simulink model "Example"  (Simulink 7.3)
settings: Solver=ode45  StartTime=10  StopTime=3600  RelTol=1e-3
libraries: simulink x2
settings Model: Creator=admin  LastModifiedBy=admin

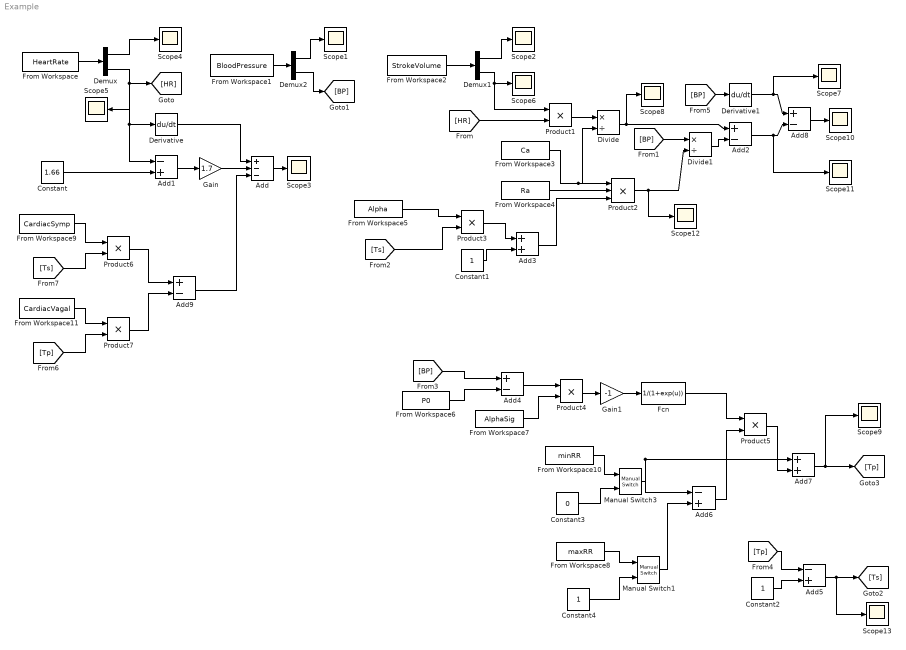
== system Example ==
  Add : Sum  Inputs=+--  OutDataType=fixdt(1, 16)  OutScaling=2^-10
  Add1 : Sum  Inputs=-+  OutDataType=fixdt(1, 16)  OutScaling=2^-10
  Add{2,4,8..9} (4 alike) : Sum  Inputs=+-  OutDataType=fixdt(1, 16)  OutScaling=2^-10
  Add3 : Sum  OutDataType=fixdt(1, 16)  OutScaling=2^-10
  Add5 : Sum  Inputs=-+  OutDataType=fixdt(1, 16)  OutScaling=2^-10
  Add6 : Sum  Inputs=-+  OutDataType=fixdt(1, 16)  OutScaling=2^-10
  Add7 : Sum  OutDataType=fixdt(1, 16)  OutScaling=2^-10
  Constant : Constant  Value=1.66  OutDataType=fixdt(1, 16)  OutScaling=2^0
  Constant1 : Constant  OutDataType=fixdt(1, 16)  OutScaling=2^0
  Constant2 : Constant  OutDataType=fixdt(1, 16)  OutScaling=2^0
  Constant3 : Constant  Value=0  OutDataType=fixdt(1, 16)  OutScaling=2^0
  Constant4 : Constant  OutDataType=fixdt(1, 16)  OutScaling=2^0
  Demux : Demux  Outputs=2
  Demux1 : Demux  Outputs=2
  Demux2 : Demux  Outputs=2
  Derivative : Derivative
  Derivative1 : Derivative
  Divide : Product  Inputs=*/  OutDataType=fixdt(1, 16)  OutScaling=2^-10
  Divide1 : Product  Inputs=*/  OutDataType=fixdt(1, 16)  OutScaling=2^-10
  Fcn : Fcn  Expr=1/(1+exp(u))
  From Workspace : FromWorkspace  VariableName=HeartRate  SampleTime=1
  From Workspace1 : FromWorkspace  VariableName=BloodPressure  SampleTime=1
  From Workspace10 : FromWorkspace  VariableName=minRR  SampleTime=0
  From Workspace11 : FromWorkspace  VariableName=CardiacVagal  SampleTime=1
  From Workspace2 : FromWorkspace  VariableName=StrokeVolume  SampleTime=1
  From Workspace3 : FromWorkspace  VariableName=Ca  SampleTime=0
  From Workspace4 : FromWorkspace  VariableName=Ra  SampleTime=0
  From Workspace5 : FromWorkspace  VariableName=Alpha  SampleTime=0
  From Workspace6 : FromWorkspace  VariableName=P0  SampleTime=0
  From Workspace7 : FromWorkspace  VariableName=AlphaSig  SampleTime=0
  From Workspace8 : FromWorkspace  VariableName=maxRR  SampleTime=0
  From Workspace9 : FromWorkspace  VariableName=CardiacSymp  SampleTime=1
  Gain : Gain  Gain=1.7  ParameterDataType=fixdt(1, 16)  ParameterScaling=2^0  OutDataType=fixdt(1, 16)  OutScaling=2^0
  Gain1 : Gain  Gain=-1  ParameterDataType=fixdt(1, 16)  ParameterScaling=2^0  OutDataType=fixdt(1, 16)  OutScaling=2^0
  Manual Switch1 : simulink/Signal Routing/Manual Switch  SystemSampleTime=-1  sw=0  action=0  varsize=off
  Manual Switch3 : simulink/Signal Routing/Manual Switch  SystemSampleTime=-1  sw=0  action=0  varsize=off
  Product{1,3..7} (6 alike) : Product  OutDataType=fixdt(1, 16)  OutScaling=2^0  RndMeth=Zero
  Product2 : Product  Inputs=3  OutDataType=fixdt(1, 16)  OutScaling=2^0  RndMeth=Zero
  Scope{1..13} (13 alike) : Scope
      Scope10 settings: SaveName=ScopeData9
      Scope11 settings: SaveName=ScopeData10
      Scope12 settings: SaveName=ScopeData11
      Scope13 settings: SaveName=ScopeData12
      Scope2 settings: SaveName=ScopeData2
      Scope3 settings: SaveName=ScopeData3
      Scope5 settings: SaveName=ScopeData5
      Scope6 settings: SaveName=ScopeData4
      Scope7 settings: SaveName=ScopeData6
      Scope8 settings: SaveName=ScopeData7
      Scope9 settings: SaveName=ScopeData8
  wires:
  From Workspace/1 -> Demux/1
  From Workspace2/1 -> Demux1/1
  Demux/1 -> Scope4/1
  Demux/2 -> Scope5/1, Derivative/1, Add1/1, [HR]
  Constant/1 -> Add1/2
  Add1/1 -> Gain/1
  Add/1 -> Scope3/1
  Demux1/2 -> Product1/1, Scope6/1
  Product1/1 -> Divide/1
  [HR] -> Product1/2
  From Workspace3/1 -> Divide/2, Product2/1
  Divide/1 -> Add2/1, Scope8/1
  Demux1/1 -> Scope2/1
  [BP] -> Divide1/1
  Product2/1 -> Divide1/2, Scope12/1
  [Ts] -> Product3/2
  Product3/1 -> Add3/1
  Constant1/1 -> Add3/2
  Add3/1 -> Product2/3
  Divide1/1 -> Add2/2
  [BP] -> Add4/1
  From Workspace6/1 -> Add4/2
  Add4/1 -> Product4/1
  From Workspace7/1 -> Product4/2
  Product4/1 -> Gain1/1
  Gain1/1 -> Fcn/1
  [Tp] -> Add5/1
  Constant2/1 -> Add5/2
  Add5/1 -> [Ts], Scope13/1
  Add2/1 -> Add8/2, Scope11/1
  [BP] -> Derivative1/1
  Derivative1/1 -> Add8/1, Scope7/1
  From Workspace1/1 -> Demux2/1
  Demux2/1 -> Scope1/1
  Demux2/2 -> [BP]
  Fcn/1 -> Product5/1
  Product5/1 -> Add7/2
  Add7/1 -> [Tp], Scope9/1
  Add6/1 -> Product5/2
  Manual Switch1/1 -> Add6/2
  From Workspace10/1 -> Manual Switch3/1
  Constant3/1 -> Manual Switch3/2
  Manual Switch3/1 -> Add6/1, Add7/1
  From Workspace8/1 -> Manual Switch1/1
  Constant4/1 -> Manual Switch1/2
  Add8/1 -> Scope10/1
  From Workspace4/1 -> Product2/2
  From Workspace9/1 -> Product6/1
  [Ts] -> Product6/2
  From Workspace11/1 -> Product7/1
  [Tp] -> Product7/2
  Product6/1 -> Add9/1
  Product7/1 -> Add9/2
  Derivative/1 -> Add/1
  Gain/1 -> Add/2
  Add9/1 -> Add/3
  From Workspace5/1 -> Product3/1
